simulink model "Simulation_based_Verification"  (R2024b)
settings: Solver=VariableStepAuto  StartTime=0.0  StopTime=0.5  RelTol=1e-3
undefined symbols (not defined in the file): D1, Delta
libraries: spsFourierLib x24, spsThreePhasePISectionLineLib x6, spsThreePhaseParallelRLCLoadLib x6, spsThreePhaseVIMeasurementLib x6, spsThreePhaseFaultLib x4, spsThreePhaseTransformerTwoWindingsLib x2, spsThreePhaseSourceLib x2, spspowerguiLib x2
settings Model: Creator=Sabyasachi  LastModifiedBy=Sabyasachi

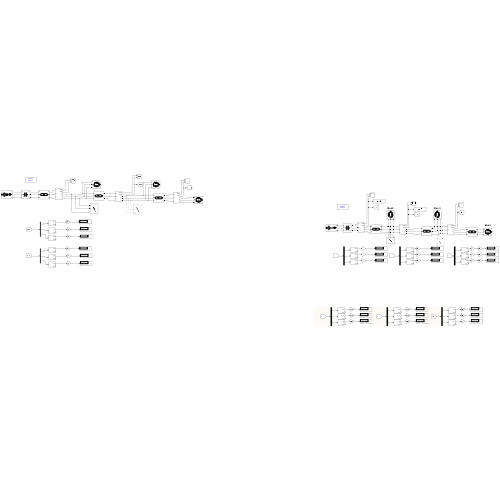
[thumbnail: Simulink's stored preview of the top-level diagram]
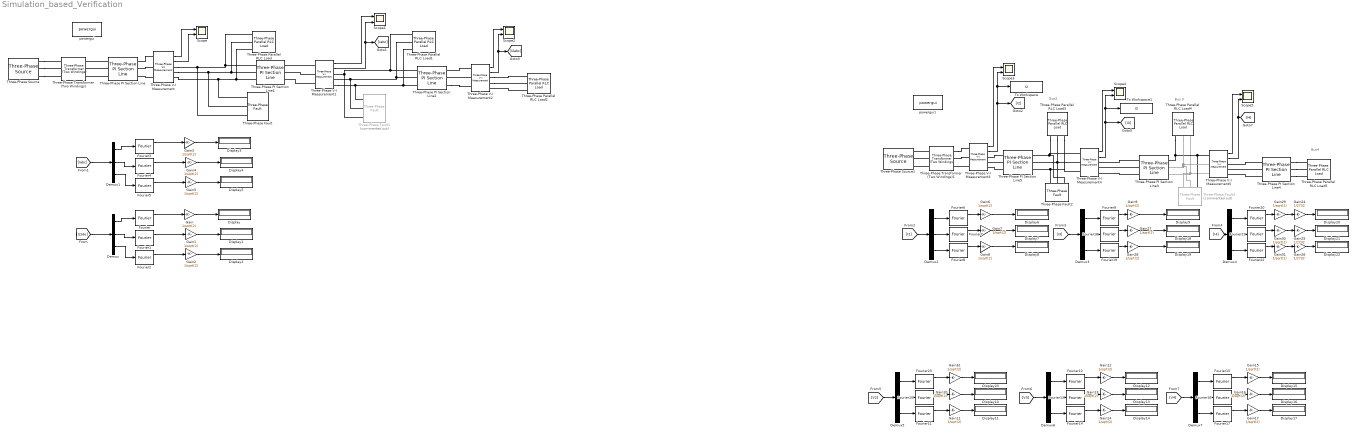
== system Simulation_based_Verification ==
  note: Bus2
  note: Bus4
  note: Bus 3
  Demux{,1..7} (8 alike) : Demux  Outputs=3
  Display{,1..23} (24 alike) : Display
  Fourier{,1..23} (24 alike) : spsFourierLib/Fourier  Freq=50  n=1  InInit=[0, 0]  Ts=0
  Gain{,1..17,27..32} (24 alike) : Gain  Gain=1/sqrt(2)
  Gain24 : Gain  Gain=1/2732
  Gain25 : Gain  Gain=1/2732
  Gain26 : Gain  Gain=1/2732
  Scope{,1..5} (6 alike) : Scope  NumInputPorts=2
  Three-Phase PI Section Line : spsThreePhasePISectionLineLib/Three-Phase PI Section Line  LConnTagsString=a|b|c  RConnTagsString=A|B|C  Length=1  Frequency=50  Resistances=[0.07 0.14]  Inductances=[ 0.07 0.14]  Capacitances=[12.74e-9 7.751e-9]
  Three-Phase PI Section Line1 : spsThreePhasePISectionLineLib/Three-Phase PI Section Line  LConnTagsString=a|b|c  RConnTagsString=A|B|C  Length=1  Frequency=50  Resistances=[0.07 0.14]  Inductances=[ 0.07 0.14]  Capacitances=[12.74e-9 7.751e-9]
  Three-Phase PI Section Line2 : spsThreePhasePISectionLineLib/Three-Phase PI Section Line  LConnTagsString=a|b|c  RConnTagsString=A|B|C  Length=100  Frequency=50  Resistances=[0.07 0.14]  Inductances=[ 0.07 0.14]  Capacitances=[12.74e-9 7.751e-9]
  Three-Phase PI Section Line3 : spsThreePhasePISectionLineLib/Three-Phase PI Section Line  LConnTagsString=a|b|c  RConnTagsString=A|B|C  Length=1  Frequency=50  Resistances=[0.1486 0.2972]  Inductances=[4.73e-4 9.46e-4]  Capacitances=[1e-12 1e-12]
  Three-Phase PI Section Line4 : spsThreePhasePISectionLineLib/Three-Phase PI Section Line  LConnTagsString=a|b|c  RConnTagsString=A|B|C  Length=1  Frequency=50  Resistances=[0.1486 0.2972]  Inductances=[4.73e-4 9.46e-4]  Capacitances=[1e-12 1e-12]
  Three-Phase PI Section Line5 : spsThreePhasePISectionLineLib/Three-Phase PI Section Line  LConnTagsString=a|b|c  RConnTagsString=A|B|C  Length=1  Frequency=50  Resistances=[0.1486 0.2972]  Inductances=[4.73e-4 9.46e-4]  Capacitances=[1e-12 1e-12]
  Three-Phase Parallel RLC Load : spsThreePhaseParallelRLCLoadLib/Three-Phase Parallel RLC Load  LConnTagsString=A|B|C  Configuration=Y (grounded)  NominalVoltage=11e3  Vabc=[1e3 1e3 1e3]  Vabcp=[1e3 1e3 1e3]  NominalFrequency=50  UnbalancedPower=off  ActivePower=2.85e6  InductivePower=100  CapacitivePower=0  Pabc=[10e3 9e3 11e3]  QLabc=[100 90 110]  QCabc=[100 90 110]  Pabcp=[10e3 9e3 11e3]  QLabcp=[100 90 110]  QCabcp=[100 90 110]  Measurements=None  LoadType=constant Z
  Three-Phase Parallel RLC Load1 : spsThreePhaseParallelRLCLoadLib/Three-Phase Parallel RLC Load  LConnTagsString=A|B|C  Configuration=Y (grounded)  NominalVoltage=11e3  Vabc=[1e3 1e3 1e3]  Vabcp=[1e3 1e3 1e3]  NominalFrequency=50  UnbalancedPower=off  ActivePower=1.90e6  InductivePower=100  CapacitivePower=0  Pabc=[10e3 9e3 11e3]  QLabc=[100 90 110]  QCabc=[100 90 110]  Pabcp=[10e3 9e3 11e3]  QLabcp=[100 90 110]  QCabcp=[100 90 110]  Measurements=None  LoadType=constant Z
  Three-Phase Parallel RLC Load2 : spsThreePhaseParallelRLCLoadLib/Three-Phase Parallel RLC Load  LConnTagsString=A|B|C  Configuration=Y (grounded)  NominalVoltage=11e3  Vabc=[1e3 1e3 1e3]  Vabcp=[1e3 1e3 1e3]  NominalFrequency=50  UnbalancedPower=off  ActivePower=3.81e6  InductivePower=100  CapacitivePower=0  Pabc=[10e3 9e3 11e3]  QLabc=[100 90 110]  QCabc=[100 90 110]  Pabcp=[10e3 9e3 11e3]  QLabcp=[100 90 110]  QCabcp=[100 90 110]  Measurements=None  LoadType=constant Z
  Three-Phase Parallel RLC Load3 : spsThreePhaseParallelRLCLoadLib/Three-Phase Parallel RLC Load  LConnTagsString=A|B|C  Configuration=Y (grounded)  NominalVoltage=11e3  Vabc=[1e3 1e3 1e3]  Vabcp=[1e3 1e3 1e3]  NominalFrequency=50  UnbalancedPower=off  ActivePower=2.42e6  InductivePower=1.245e6  CapacitivePower=0  Pabc=[10e3 9e3 11e3]  QLabc=[100 90 110]  QCabc=[100 90 110]  Pabcp=[10e3 9e3 11e3]  QLabcp=[100 90 110]  QCabcp=[100 90 110]  Measurements=None  LoadType=constant Z
  Three-Phase Parallel RLC Load4 : spsThreePhaseParallelRLCLoadLib/Three-Phase Parallel RLC Load  LConnTagsString=A|B|C  Configuration=Y (grounded)  NominalVoltage=11e3  Vabc=[1e3 1e3 1e3]  Vabcp=[1e3 1e3 1e3]  NominalFrequency=50  UnbalancedPower=off  ActivePower=1.61e6  InductivePower=0.830e6  CapacitivePower=0  Pabc=[10e3 9e3 11e3]  QLabc=[100 90 110]  QCabc=[100 90 110]  Pabcp=[10e3 9e3 11e3]  QLabcp=[100 90 110]  QCabcp=[100 90 110]  Measurements=None  LoadType=constant Z
  Three-Phase Parallel RLC Load5 : spsThreePhaseParallelRLCLoadLib/Three-Phase Parallel RLC Load  LConnTagsString=A|B|C  Configuration=Y (grounded)  NominalVoltage=11e3  Vabc=[1e3 1e3 1e3]  Vabcp=[1e3 1e3 1e3]  NominalFrequency=50  UnbalancedPower=off  ActivePower=3.23e6  InductivePower=1.660e6  CapacitivePower=0  Pabc=[10e3 9e3 11e3]  QLabc=[100 90 110]  QCabc=[100 90 110]  Pabcp=[10e3 9e3 11e3]  QLabcp=[100 90 110]  QCabcp=[100 90 110]  Measurements=None  LoadType=constant Z
  Three-Phase Transformer (Two Windings) : spsThreePhaseTransformerTwoWindingsLib/Three-Phase Transformer (Two Windings)  Winding1Connection=Delta (D1)  Winding2Connection=Yg  CoreType=Three single-phase transformers  SetSaturation=off  Hysteresis=off  DataFile='hysteresis'  SetInitialFlux=off  Measurements=None  UNITS=pu  NominalPower=[ 17e6 , 50 ]  Winding1=[ 33e3 , 0.002 , 0.05 ]  Winding2=[ 11e3 , 0.002 , 0.05 ]  Rm=500  Lm=500  L0=0.5  Saturation=[ 0,0 ; 0.0024,1.2 ; 1.0,1.52 ]  InitialFluxes=[ 0.8 , -0.8 , 0.7 ]  BreakLoop=off  DiscreteSolver=Trapezoidal iterative  DataType=off  TransfoNumber=1
  Three-Phase Transformer (Two Windings)1 : spsThreePhaseTransformerTwoWindingsLib/Three-Phase Transformer (Two Windings)  Winding1Connection=Delta (D1)  Winding2Connection=Yg  CoreType=Three single-phase transformers  SetSaturation=off  Hysteresis=off  DataFile='hysteresis'  SetInitialFlux=off  Measurements=None  UNITS=pu  NominalPower=[ 17e6 , 50 ]  Winding1=[33e3 , 1e-6 , 0.05 ]  Winding2=[ 11e3 , 1e-6 , 1e-6 ]  Rm=500  Lm=500  L0=0.5  Saturation=[ 0,0 ; 0.0024,1.2 ; 1.0,1.52 ]  InitialFluxes=[ 0.8 , -0.8 , 0.7 ]  BreakLoop=off  DiscreteSolver=Trapezoidal iterative  DataType=off  TransfoNumber=1
  Three-Phase V-I Measurement{,1..5} (6 alike) : spsThreePhaseVIMeasurementLib/Three-Phase V-I Measurement  VoltageMeasurement=phase-to-ground  SetLabelV=off  LabelV=Vabc  Vpu=off  VpuLL=off  CurrentMeasurement=yes  SetLabelI=off  LabelI=Iabc  Ipu=off  Pbase=100e6  Vbase=500e3  OutputType=Complex  PhasorSimulation=off  PSBequivalent=0
  Three-Phase Fault : spsThreePhaseFaultLib/Three-Phase Fault  InitialStates=0  FaultA=on  FaultB=on  FaultC=on  GroundFault=on  SwitchTimes="[0.15  0.25]"  External=off  SwitchStatus=NaN  FaultResistance=0.001  GroundResistance=0.01  SnubberResistance=1e6  SnubberCapacitance=inf  Measurements=None
  Three-Phase Fault1 : spsThreePhaseFaultLib/Three-Phase Fault  Commented=on  InitialStates=0  FaultA=on  FaultB=off  FaultC=off  GroundFault=on  SwitchTimes="[0.3  0.4]"  External=off  SwitchStatus=NaN  FaultResistance=0.001  GroundResistance=0.01  SnubberResistance=1e6  SnubberCapacitance=inf  Measurements=None
  Three-Phase Fault2 : spsThreePhaseFaultLib/Three-Phase Fault  InitialStates=0  FaultA=on  FaultB=on  FaultC=on  GroundFault=on  SwitchTimes=[0.2]  External=off  SwitchStatus=NaN  FaultResistance=0.001  GroundResistance=0.01  SnubberResistance=1e6  SnubberCapacitance=inf  Measurements=None
  Three-Phase Fault3 : spsThreePhaseFaultLib/Three-Phase Fault  Commented=on  InitialStates=0  FaultA=on  FaultB=off  FaultC=off  GroundFault=on  SwitchTimes=[0.2]  External=off  SwitchStatus=NaN  FaultResistance=0.001  GroundResistance=0.01  SnubberResistance=1e6  SnubberCapacitance=inf  Measurements=None
  Three-Phase Source : spsThreePhaseSourceLib/Three-Phase Source  InternalConnection=Yg  VoltagePhases=off  Voltage=33e3  PhaseAngle=0  Voltage_phases=[25e3 25e3 25e3]/sqrt(3)  PhaseAngles_phases=[0 -120 +120]  Frequency=50  NonIdealSource=on  SpecifyImpedance=off  Resistance=0.8929  Inductance=16.58e-3  ShortCircuitLevel=100e6  BaseVoltage=25e3  XRratio=7  BusType=swing  Pref=10e3  Qref=0  Prefabc=[10e3, 10e3, 10e3]  Qrefabc=[0, 0, 0]  Qmin=-inf  Qmax=inf
  Three-Phase Source1 : spsThreePhaseSourceLib/Three-Phase Source  InternalConnection=Yg  VoltagePhases=off  Voltage=33e3  PhaseAngle=0  Voltage_phases=[25e3 25e3 25e3]/sqrt(3)  PhaseAngles_phases=[0 -120 +120]  Frequency=50  NonIdealSource=on  SpecifyImpedance=off  Resistance=0  Inductance=0.01  ShortCircuitLevel=100e6  BaseVoltage=33e3  XRratio=7  BusType=swing  Pref=10e3  Qref=0  Prefabc=[10e3, 10e3, 10e3]  Qrefabc=[0, 0, 0]  Qmin=-inf  Qmax=inf
  To Workspace : ToWorkspace  VariableName=I2  SaveFormat=Timeseries  SampleTime=-1
  To Workspace1 : ToWorkspace  VariableName=I3  SaveFormat=Timeseries  SampleTime=-1
  powergui : spspowerguiLib/powergui  Priority=1  SimulationMode=Discrete  SampleTime=50e-6  frequency=60  Iterations=50  frequencyindice=50  Pbase=100e6  ErrMax=1e-4  UnitsV=kV  UnitsW=MW  buscounter=0  FunctionMessages=off  echomessages=off  EnableUseOfTLC=off  CurrentSourceSwitches=off  DisableSnubberDevices=off  DisableRonSwitches=off  DisableVfSwitches=off  DisplayEquations=off  AutomaticDiscreteSolvers=off  SolverType=Tustin/Backward Euler (TBE)  Interpol=off  ExternalGateDelay=off  methode=off  Ts=100  x0status=blocks  SPID=on  SwTol=0  HookPort=off  NonlinearTolerance=1e-4  nMaxIteration=100  ContinueOnMaxIteration=off  RestoreLinks=warning  ResistiveCurrentMeasurement=off  Frange=[0:2:500]  Ylog=off  Xlog=on  ShowGrid=off  save=off  variable=ZData  structure=0  ZoomFFT=off  StartTime=0.0  cycles=1  DisplayStyle=1  fundamental=60  FreqAxis=off  MaxFrequency=1000  frequencyindicesteady=1  RmsSteady=1  display=off
  powergui1 : spspowerguiLib/powergui  Priority=1  SimulationMode=Discrete  SampleTime=50e-6  frequency=50  Iterations=50  frequencyindice=50  Pbase=100e6  ErrMax=1e-4  UnitsV=kV  UnitsW=MW  buscounter=0  FunctionMessages=off  echomessages=off  EnableUseOfTLC=off  CurrentSourceSwitches=off  DisableSnubberDevices=off  DisableRonSwitches=off  DisableVfSwitches=off  DisplayEquations=off  AutomaticDiscreteSolvers=off  SolverType=Tustin/Backward Euler (TBE)  Interpol=off  ExternalGateDelay=off  methode=off  Ts=100  x0status=blocks  SPID=on  SwTol=0  HookPort=off  NonlinearTolerance=1e-4  nMaxIteration=100  ContinueOnMaxIteration=off  RestoreLinks=warning  ResistiveCurrentMeasurement=off  Frange=[0:2:500]  Ylog=off  Xlog=on  ShowGrid=off  save=off  variable=ZData  structure=0  ZoomFFT=off  StartTime=0.0  cycles=1  DisplayStyle=1  fundamental=60  FreqAxis=off  MaxFrequency=1000  frequencyindicesteady=1  RmsSteady=1  display=off
  wires:
  Three-Phase V-I Measurement/1 -> Scope/1
  Three-Phase V-I Measurement/2 -> Scope/2
  Three-Phase V-I Measurement1/1 -> Scope1/1
  Three-Phase V-I Measurement1/2 -> [Iabc], Scope1/2
  Three-Phase V-I Measurement2/1 -> Scope2/1
  [I2abc] -> Demux/1
  Demux/2 -> Fourier1/1
  Fourier1/1 -> Gain1/1
  Gain1/1 -> Display1/1
  Gain/1 -> Display/1
  Fourier2/1 -> Gain2/1
  Demux/1 -> Fourier/1
  Gain2/1 -> Display2/1
  Fourier/1 -> Gain/1
  Demux/3 -> Fourier2/1
  Demux1/3 -> Fourier5/1
  Fourier3/1 -> Gain3/1
  Gain5/1 -> Display5/1
  Demux1/1 -> Fourier3/1
  Fourier5/1 -> Gain5/1
  Gain3/1 -> Display3/1
  Gain4/1 -> Display4/1
  Fourier4/1 -> Gain4/1
  Demux1/2 -> Fourier4/1
  [Iabc] -> Demux1/1
  Three-Phase V-I Measurement2/2 -> [I2abc], Scope2/2
  Three-Phase V-I Measurement3/1 -> Scope3/1
  Three-Phase V-I Measurement5/2 -> Scope5/2, [I4]
  Three-Phase V-I Measurement4/1 -> Scope4/1
  Three-Phase V-I Measurement5/1 -> Scope5/1
  Three-Phase V-I Measurement3/2 -> To Workspace/1, Scope3/2, [I2]
  Three-Phase V-I Measurement4/2 -> Scope4/2, To Workspace1/1, [I3]
  Demux5/2 -> Fourier10/1
  Demux6/2 -> Fourier13/1
  Demux3/1 -> Fourier9/1
  Gain7/1 -> Display7/1
  Demux5/3 -> Fourier11/1
  [I2] -> Demux2/1
  Fourier17/1 -> Gain17/1
  Fourier23/1 -> Gain32/1
  Gain17/1 -> Display17/1
  Gain8/1 -> Display8/1
  Fourier18/1 -> Gain27/1
  Demux6/1 -> Fourier12/1
  Fourier13/1 -> Gain13/1
  Fourier22/1 -> Gain31/1
  Gain26/1 -> Display22/1
  Gain32/1 -> Display23/1
  Demux4/3 -> Fourier22/1
  Gain27/1 -> Display18/1
  Fourier14/1 -> Gain14/1
  Demux2/2 -> Fourier7/1
  Fourier19/1 -> Gain28/1
  Gain30/1 -> Gain25/1
  Gain11/1 -> Display11/1
  [V3] -> Demux6/1
  Fourier9/1 -> Gain9/1
  Gain9/1 -> Display9/1
  [V4] -> Demux7/1
  Fourier21/1 -> Gain30/1
  Fourier8/1 -> Gain8/1
  Demux7/3 -> Fourier17/1
  Gain25/1 -> Display21/1
  Gain31/1 -> Gain26/1
  Gain24/1 -> Display20/1
  [I4] -> Demux4/1
  [I3] -> Demux3/1
  Fourier20/1 -> Gain29/1
  Fourier7/1 -> Gain7/1
  Demux3/3 -> Fourier19/1
  Demux7/2 -> Fourier16/1
  Gain28/1 -> Display19/1
  Demux3/2 -> Fourier18/1
  Gain29/1 -> Gain24/1
  Demux2/3 -> Fourier8/1
  Fourier12/1 -> Gain12/1
  Gain14/1 -> Display14/1
  Demux4/1 -> Fourier20/1
  Demux5/1 -> Fourier23/1
  Fourier15/1 -> Gain15/1
  Gain15/1 -> Display15/1
  Fourier16/1 -> Gain16/1
  Gain12/1 -> Display12/1
  Fourier11/1 -> Gain11/1
  Gain10/1 -> Display10/1
  Demux2/1 -> Fourier6/1
  Demux7/1 -> Fourier15/1
  Fourier10/1 -> Gain10/1
  Demux4/2 -> Fourier21/1
  [V2] -> Demux5/1
  Gain16/1 -> Display16/1
  Demux6/3 -> Fourier14/1
  Gain13/1 -> Display13/1
  Gain6/1 -> Display6/1
  Fourier6/1 -> Gain6/1
  connections:
  Three-Phase Source/RConn1 -- Three-Phase Transformer (Two Windings)/LConn1
  Three-Phase Source/RConn2 -- Three-Phase Transformer (Two Windings)/LConn2
  Three-Phase Source/RConn3 -- Three-Phase Transformer (Two Windings)/LConn3
  Three-Phase PI Section Line/LConn1 -- Three-Phase Transformer (Two Windings)/RConn1
  Three-Phase PI Section Line/LConn2 -- Three-Phase Transformer (Two Windings)/RConn2
  Three-Phase PI Section Line/LConn3 -- Three-Phase Transformer (Two Windings)/RConn3
  Three-Phase V-I Measurement/LConn2 -- Three-Phase PI Section Line/RConn2
  Three-Phase V-I Measurement/LConn3 -- Three-Phase PI Section Line/RConn3
  Three-Phase V-I Measurement/LConn1 -- Three-Phase PI Section Line/RConn1
  Three-Phase V-I Measurement1/LConn1 -- Three-Phase PI Section Line1/RConn1
  Three-Phase V-I Measurement1/LConn2 -- Three-Phase PI Section Line1/RConn2
  Three-Phase V-I Measurement1/LConn3 -- Three-Phase PI Section Line1/RConn3
  Three-Phase V-I Measurement2/LConn2 -- Three-Phase PI Section Line2/RConn2
  Three-Phase V-I Measurement2/LConn1 -- Three-Phase PI Section Line2/RConn1
  Three-Phase PI Section Line2/RConn3 -- Three-Phase V-I Measurement2/LConn3
  Three-Phase PI Section Line2/LConn1 -- Three-Phase Parallel RLC Load1/LConn1 -- Three-Phase Fault1/LConn3 -- Three-Phase V-I Measurement1/RConn1
  Three-Phase PI Section Line2/LConn2 -- Three-Phase Parallel RLC Load1/LConn2 -- Three-Phase Fault1/LConn2 -- Three-Phase V-I Measurement1/RConn2
  Three-Phase V-I Measurement1/RConn3 -- Three-Phase Fault1/LConn1 -- Three-Phase Parallel RLC Load1/LConn3 -- Three-Phase PI Section Line2/LConn3
  Three-Phase V-I Measurement/RConn1 -- Three-Phase Fault/LConn3 -- Three-Phase Parallel RLC Load/LConn1 -- Three-Phase PI Section Line1/LConn1
  Three-Phase V-I Measurement/RConn2 -- Three-Phase Fault/LConn2 -- Three-Phase Parallel RLC Load/LConn2 -- Three-Phase PI Section Line1/LConn2
  Three-Phase V-I Measurement/RConn3 -- Three-Phase Fault/LConn1 -- Three-Phase Parallel RLC Load/LConn3 -- Three-Phase PI Section Line1/LConn3
  Three-Phase Parallel RLC Load2/LConn3 -- Three-Phase V-I Measurement2/RConn3
  Three-Phase V-I Measurement2/RConn2 -- Three-Phase Parallel RLC Load2/LConn2
  Three-Phase V-I Measurement2/RConn1 -- Three-Phase Parallel RLC Load2/LConn1
  Three-Phase V-I Measurement4/LConn1 -- Three-Phase PI Section Line5/RConn1 -- Three-Phase Parallel RLC Load3/LConn1 -- Three-Phase Fault2/LConn1
  Three-Phase Fault3/LConn3 -- Three-Phase PI Section Line3/RConn3 -- Three-Phase Parallel RLC Load4/LConn3 -- Three-Phase V-I Measurement5/LConn3
  Three-Phase V-I Measurement5/LConn1 -- Three-Phase PI Section Line3/RConn1 -- Three-Phase Parallel RLC Load4/LConn1 -- Three-Phase Fault3/LConn1
  Three-Phase Fault3/LConn2 -- Three-Phase Parallel RLC Load4/LConn2 -- Three-Phase V-I Measurement5/LConn2 -- Three-Phase PI Section Line3/RConn2
  Three-Phase Fault2/LConn3 -- Three-Phase PI Section Line5/RConn3 -- Three-Phase Parallel RLC Load3/LConn3 -- Three-Phase V-I Measurement4/LConn3
  Three-Phase Fault2/LConn2 -- Three-Phase PI Section Line5/RConn2 -- Three-Phase Parallel RLC Load3/LConn2 -- Three-Phase V-I Measurement4/LConn2
  Three-Phase PI Section Line3/LConn2 -- Three-Phase V-I Measurement4/RConn2
  Three-Phase V-I Measurement3/LConn2 -- Three-Phase Transformer (Two Windings)1/RConn2
  Three-Phase PI Section Line4/RConn2 -- Three-Phase Parallel RLC Load5/LConn2
  Three-Phase Transformer (Two Windings)1/LConn1 -- Three-Phase Source1/RConn1
  Three-Phase Transformer (Two Windings)1/LConn3 -- Three-Phase Source1/RConn3
  Three-Phase PI Section Line4/LConn2 -- Three-Phase V-I Measurement5/RConn2
  Three-Phase PI Section Line4/RConn1 -- Three-Phase Parallel RLC Load5/LConn1
  Three-Phase PI Section Line3/LConn1 -- Three-Phase V-I Measurement4/RConn1
  Three-Phase Transformer (Two Windings)1/RConn1 -- Three-Phase V-I Measurement3/LConn1
  Three-Phase PI Section Line4/RConn3 -- Three-Phase Parallel RLC Load5/LConn3
  Three-Phase PI Section Line4/LConn1 -- Three-Phase V-I Measurement5/RConn1
  Three-Phase Transformer (Two Windings)1/LConn2 -- Three-Phase Source1/RConn2
  Three-Phase PI Section Line3/LConn3 -- Three-Phase V-I Measurement4/RConn3
  Three-Phase PI Section Line4/LConn3 -- Three-Phase V-I Measurement5/RConn3
  Three-Phase V-I Measurement3/LConn3 -- Three-Phase Transformer (Two Windings)1/RConn3
  Three-Phase PI Section Line5/LConn1 -- Three-Phase V-I Measurement3/RConn1
  Three-Phase PI Section Line5/LConn2 -- Three-Phase V-I Measurement3/RConn2
  Three-Phase PI Section Line5/LConn3 -- Three-Phase V-I Measurement3/RConn3
